simulink model "Simulation"  (R2024b)
settings: Solver=VariableStepAuto  StartTime=0.0  StopTime=600  RelTol=1e-3
values from neighbouring files (symbols this model uses):
  H = [0 40 60 70 80 250]    [Params.m]
  I_ideal = 20    [Params.m]
  K1 = 1    [Params.m]
  magazzino_diametri = [430 320 260 230 540]    [Params.m]
  magazzino_legno = [1 5 2 4 3]    [Params.m]
  tau = 0.5    [Params.m]
  wood = [0 1 2 3 4 5]    [Params.m]
libraries: simulink x1, slpidlib x1
settings Model: Creator=eliasantuari  LastModifiedBy=eliasantuari

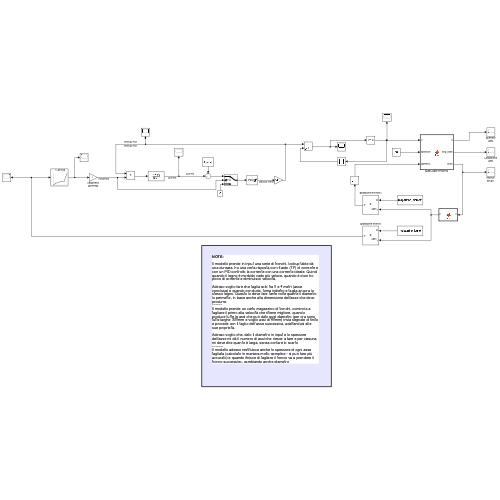
[thumbnail: Simulink's stored preview of the top-level diagram]
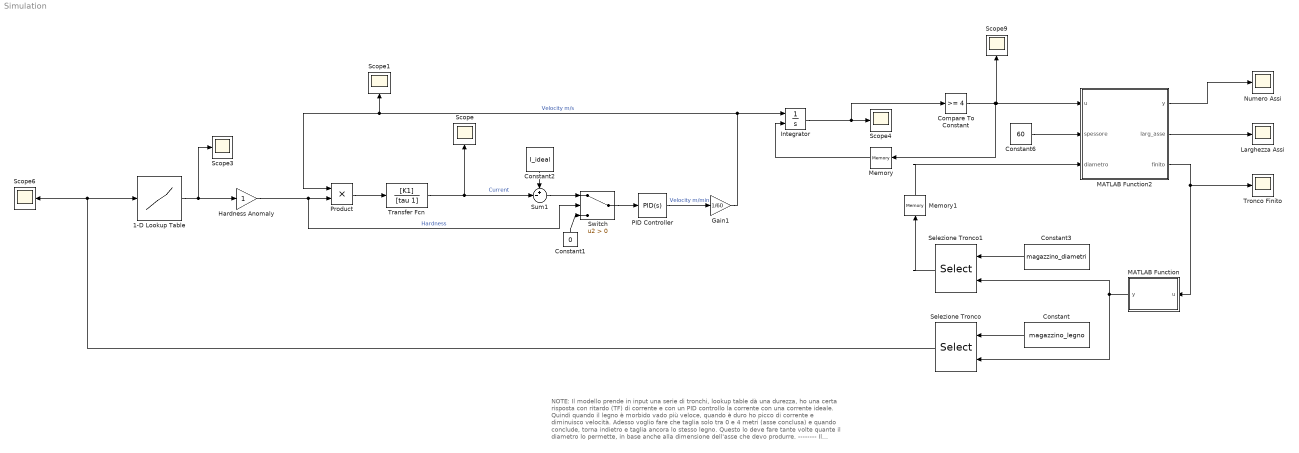
== system Simulation ==
  note: NOTE:
      |
      | Il modello prende in input una serie di tronchi, lookup table dà una durezza, ho una certa risposta con ritardo (TF) di corrente e con un PID controllo la corrente con una corrente ideale. Quindi quando il legno è morbido vado più veloce, quando è duro ho picco di corrente e diminuisco velocità.
      |
      | Adesso voglio fare che taglia solo tra 0 e 4 metri (asse conclusa) e quando conclude, torna indietro e taglia ancora lo stesso legno. Questo lo deve fare tante volte quante il diametro lo permette, in base anche alla dimensione dell'asse che devo produrre.
      | --------
      | Il modello prende un certo magazzino di tronchi, comincia a tagliare il primo alla velocità che ritiene migliore, quando produce tutte le assi che può dato quel diametro (per ora sono tutte larghe 320mm e voglio assi di 60mm) invia segnale di finito e procede con il taglio dell'asse successiva, adattandosi alle sue proprietà.
      |
      | Adesso voglio che, dato il diametro in input e lo spessore dell'asse mi dà il numero di assi che riesce a fare e per ciasuna mi deve dire quanto è larga, senza contare lo scarto
      | ---------
      | Il modello adesso restituisce anche lo spessore di ogni asse tagliata (calcolato in maniera molto semplice - si può fare più accurato) e quando finisce di tagliare il tronco va a prendere il tronco successivo, cambiando anche diametro
  1-D Lookup Table : Lookup_n-D  NumberOfTableDimensions=1  BreakpointsForDimension1=wood  Table=H  InternalRulePriority=Speed  RndMeth=Simplest
  Compare To Constant : simulink/Logic and Bit Operations/Compare To Constant  relop=>=  const=4  OutDataTypeStr=boolean
  Constant : Constant  Value=magazzino_legno
  Constant1 : Constant  Value=0
  Constant2 : Constant  Value=I_ideal
  Constant3 : Constant  Value=magazzino_diametri
  Constant6 : Constant  Value=60
  Gain1 : Gain  Gain=1/60
  Hardness Anomaly : Gain
  Integrator : Integrator  ExternalReset=rising
  Larghezza Assi : Scope
  MATLAB Function : MATLAB Function  TreatAsAtomicUnit=on
  MATLAB Function2 : MATLAB Function  TreatAsAtomicUnit=on
  Memory : Memory
  Memory1 : Memory
  Numero Assi : Scope
  PID Controller : slpidlib/PID Controller  Controller=PID  Form=Parallel  TimeDomain=Continuous-time  UseExternalTs=off  SampleTime=-1  IntegratorMethod=Forward Euler  FilterMethod=Forward Euler  ControllerParametersSource=internal  P=1  I=1  UseKiTs=off  D=0  UseExternalDerivativeSource=off  N=0  UseFilter=on  TunerSelectOption=Transfer Function Based (PID Tuner App)  InitialConditionSource=internal  InitialConditionForIntegrator=0  InitialConditionForFilter=0  DifferentiatorICPrevScaledInput=0  ExternalReset=none  TrackingMode=off  Kt=1  LimitOutput=on  SatLimitsSource=internal  UpperSaturationLimit=45  LowerSaturationLimit=0  LinearizeAsGain=on  AntiWindupMode=none  Kb=1  LimitIntegrator=off  UpperIntegratorSaturationLimit=inf  LowerIntegratorSaturationLimit=-inf  POutMin=[]  POutMax=[]  IOutMin=[]  IOutMax=[]  DOutMin=[]  DOutMax=[]  NOutMin=[]  NOutMax=[]  SumOutMin=[]  SumOutMax=[]  SaturationOutMin=[]  SaturationOutMax=[]  PParamMin=[]  PParamMax=[]  IParamMin=[]  IParamMax=[]  DParamMin=[]  DParamMax=[]  NParamMin=[]  NParamMax=[]  KbParamMin=[]  KbParamMax=[]  KtParamMin=[]  KtParamMax=[]  KbOutMin=[]  KbOutMax=[]  KtOutMin=[]  KtOutMax=[]  IntegratorOutMin=[]  IntegratorOutMax=[]  FilterOutMin=[]  FilterOutMax=[]  SumI1OutMin=[]  SumI1OutMax=[]  SumI2OutMin=[]  SumI2OutMax=[]  SumI3OutMin=[]  SumI3OutMax=[]  SumI4OutMin=[]  SumI4OutMax=[]  SumDOutMin=[]  SumDOutMax=[]  DifferentiatorOutMin=[]  DifferentiatorOutMax=[]  FilterDiffOutCoefMin=[]  FilterDiffOutCoefMax=[]  ReciprocalOutMin=[]  ReciprocalOutMax=[]  SumDenOutMin=[]  SumDenOutMax=[]  SumNumOutMin=[]  SumNumOutMax=[]  DivideOutMin=[]  DivideOutMax=[]  UdiffTsProdOutMin=[]  UdiffTsProdOutMax=[]  NTsProdOutMin=[]  NTsProdOutMax=[]  UintegralTsProdOutMin=[]  UintegralTsProdOutMax=[]  UngainTsProdOutMin=[]  UngainTsProdOutMax=[]  ClampingZeroOutDataTypeStr=Inherit: Inherit via back propagation  ClampingZeroOutMin=[]  ClampingZeroOutMax=[]  FilterDenConstantOutDataTypeStr=Inherit: Inherit via back propagation  FilterDenConstantOutMin=[]  FilterDenConstantOutMax=[]  PCopyOutDataTypeStr=Inherit: Inherit via back propagation  PCopyOutMin=[]  PCopyOutMax=[]  NCopyOutDataTypeStr=Inherit: Inherit via back propagation  NCopyOutMin=[]  NCopyOutMax=[]  IntegratorContinuousStateAttributes=''  IntegratorStateMustResolveToSignalObject=off  IntegratorRTWStateStorageClass=Auto  FilterContinuousStateAttributes=''  FilterStateMustResolveToSignalObject=off  FilterRTWStateStorageClass=Auto  ParallelPVariant=InternalParameters  IdealPVariant=Disabled  IVariant=InternalParameters  DVariant=InternalParameters  IntegratorVariant=Continuous  SatVariant=Enabled  AWVariant=Passthrough  PCopyVariant=Disabled  TRVariant=Disabled  FdbkBlocksVariant=Forward  IdealPFdbkVariant=Disabled  SatFdbkVariant=Disabled  DerivativeFilterVariant=ContFilter  NVariant=InternalParameters  NCopyVariant=Disabled  FilterICVariant=InternalICsFilter  IntegratorICVariant=InternalICs  ExternalResetVariant=Disabled  TRSumVariant=Passthrough  SumFdbkVariant=Disabled  SumVariant=Sum_PID  TsampFilterVariant=InternalTs  TsampNgainVariant=Passthrough  TsampIntegralVariant=Disabled_SignalSpec  ExternalSaturationOutDataTypeStr=Inherit: Same as second input  DerivativeSourceVariant=ErrorSignal  PreIntVariant=InternalPreInt
  Product : Product
  Scope{,1,3..4,6,9} (6 alike) : Scope
  Selezione Tronco : Selector  InputPortWidth=length(magazzino_legno)  IndexOptions=Index vector (port)  Indices=[1 3]  OutputSizes=1
  Selezione Tronco1 : Selector  InputPortWidth=length(magazzino_diametri)  IndexOptions=Index vector (port)  Indices=[1 3]  OutputSizes=1
  Sum1 : Sum  Inputs=+-|
  Switch : Switch  Criteria=u2 > Threshold  SaturateOnIntegerOverflow=off  InputSameDT=off
  Transfer Fcn : TransferFcn  Numerator=[K1]  Denominator=[tau 1]
  "Tronco Finito " : Scope
  wires:
  1-D Lookup Table/1 -> Scope3/1, Hardness Anomaly/1
  Hardness Anomaly/1 -> Switch/2, Product/2  "Hardness"
  Product/1 -> Transfer Fcn/1
  PID Controller/1 -> Gain1/1  "Velocity m/min"
  Constant2/1 -> Sum1/1
  Selezione Tronco/1 -> 1-D Lookup Table/1, Scope6/1
  Switch/1 -> PID Controller/1
  Constant1/1 -> Switch/3
  Sum1/1 -> Switch/1
  Transfer Fcn/1 -> Sum1/2, Scope/1  "Current"
  Gain1/1 -> Product/1, Scope1/1, Integrator/1  "Velocity m/s"
  Integrator/1 -> Compare To Constant/1, Scope4/1
  Compare To Constant/1 -> MATLAB Function2/1(u), Scope9/1, Memory/1
  MATLAB Function2/1(y) -> Numero Assi/1
  Memory/1 -> Integrator/2
  Selezione Tronco1/1 -> Memory1/1
  Constant6/1 -> MATLAB Function2/2(spessore)
  MATLAB Function/1(y) -> Selezione Tronco1/2, Selezione Tronco/2
  Constant/1 -> Selezione Tronco/1
  MATLAB Function2/2(larg_asse) -> Larghezza Assi/1
  MATLAB Function2/3(finito) -> MATLAB Function/1(u), "Tronco Finito "/1
  Constant3/1 -> Selezione Tronco1/1
  Memory1/1 -> MATLAB Function2/3(diametro)

== matlab function Simulation/MATLAB Function ==
  data: u input; y output
function y = fcn(u)
    persistent counter
    if isempty(counter)
        counter = 1;
    end

    if u == 1
        counter = counter + 1;
    end

    
    y = counter;
end

== matlab function Simulation/MATLAB Function2 ==
  data: u input; y output; larg_asse output; spessore input; finito output; diametro input
function [y, larg_asse, finito]= fcn(u, spessore, diametro)
    persistent counter 

    max_assi = floor(diametro / spessore);
    finito = 0;
    

    if isempty(counter)
        counter = 0;
    end

    % Conto assi tagliate
    if u == 1
        counter = counter + 1;
    end

    % Quando finisco tronco segnalo e azzero counter
    if counter > max_assi
        finito = 1;
        counter = 0;
    end

    % Calcolo larghezza delle assi
    distanza_bordo = counter * spessore;
    h = abs(diametro/2 - distanza_bordo + (spessore/2));
    
    if counter == 0
        larg_asse = 0;
    else
        larg_asse = 2 * sqrt((diametro/2)^2-h^2);
    end

    y = counter;
end
